simulink model "operationalSpaceInverseDynamicsControl"  (R2021a)
settings: Solver=VariableStepAuto  StartTime=0.0  StopTime=25  RelTol=1e-3
values from neighbouring files (symbols this model uses):
  Kd = diag([100, 100, 100, 50, 50, 50])    [assignment10_main.m]
  Kp = 5*diag([100, 100, 100,50,50,50])    [assignment10_main.m]
  x_d_const = [-0.139961 ... (first row only)    [assignment10_main.m]
libraries: vrlib x1, robotcorelib x1
settings Model: Creator=fabio  LastModifiedBy=fabio

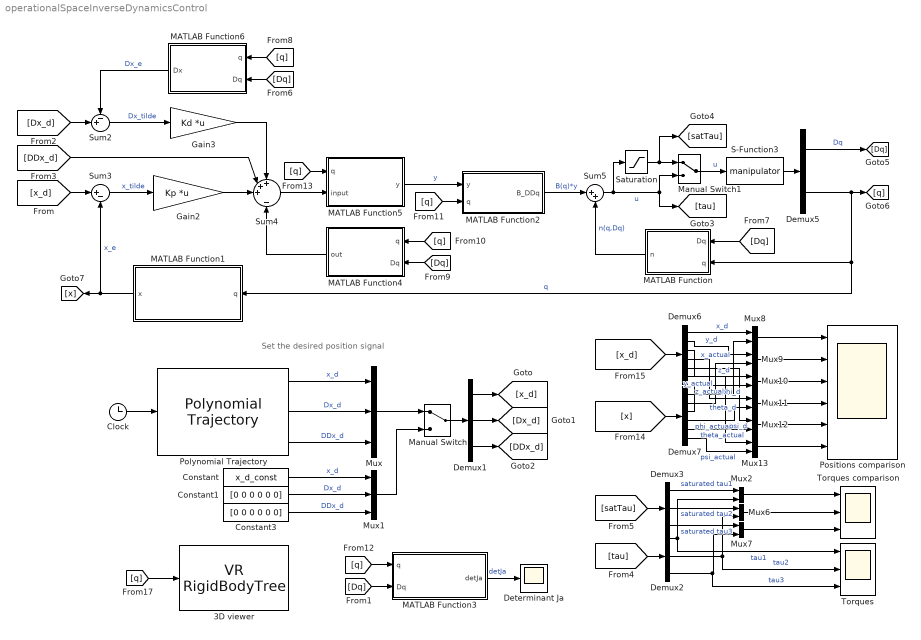
== system operationalSpaceInverseDynamicsControl ==
  note: Set the desired position signal
  3D viewer : vrlib/VR RigidBodyTree  RBT=robot  useRBT=off  Ts=0.5  ForceViewerOpen=on
      settings: SourceProductBaseCode=SL
  Clock : Clock
  Constant : Constant  Value=x_d_const
  Constant1 : Constant  Value=[0 0 0 0 0 0]
  Constant3 : Constant  Value=[0 0 0 0 0 0]
  Demux1 : Demux  Outputs=3
  Demux2 : Demux  Outputs=3
  Demux3 : Demux  Outputs=3
  Demux5 : Demux  Outputs=[3 3]
  Demux6 : Demux  Outputs=6
  Demux7 : Demux  Outputs=6
  Determinant Ja : Scope
  Gain2 : Gain  Gain=Kp  Multiplication=Matrix(K*u) (u vector)
  Gain3 : Gain  Gain=Kd  Multiplication=Matrix(K*u) (u vector)
  MATLAB Function : MATLAB Function  TreatAsAtomicUnit=on
  MATLAB Function1 : MATLAB Function  TreatAsAtomicUnit=on
  MATLAB Function2 : MATLAB Function  TreatAsAtomicUnit=on
  MATLAB Function3 : MATLAB Function  TreatAsAtomicUnit=on
  MATLAB Function4 : MATLAB Function  TreatAsAtomicUnit=on
  MATLAB Function5 : MATLAB Function  TreatAsAtomicUnit=on
  MATLAB Function6 : MATLAB Function  TreatAsAtomicUnit=on
  Manual Switch : ManualSwitch
  Manual Switch1 : ManualSwitch
  Mux : Mux  Inputs=3
  Mux1 : Mux  Inputs=3
  Mux{2,6..13} (9 alike) : Mux  Inputs=2
  Polynomial Trajectory : robotcorelib/Polynomial Trajectory  WaypointSource=Internal  Waypoints=x_d  TimePoints=[ 0, 10, 20]  TimeInterval=[ 1, 4 ]  Method=Cubic Polynomial  ParameterSource=Internal  VelocityBoundaryCondition=zeros( 6, 3)  AccelerationBoundaryCondition=zeros( 6, 3)  SimulateUsing=Interpreted execution
  Positions comparison : Scope  NumInputPorts=6
  S-Function3 : S-Function  FunctionName=manipulator  Parameters=myRobot  SFunctionDeploymentMode=off  EnableBusSupport=off
  Saturation : Saturate  UpperLimit=20  LowerLimit=-20
  Sum2 : Sum  Inputs=-+|
  Sum3 : Sum  Inputs=|+-
  Sum4 : Sum  Inputs=+++|-
  Sum5 : Sum  Inputs=|++
  Torques : Scope  NumInputPorts=3
  Torques comparison : Scope  NumInputPorts=3
  wires:
  Manual Switch1/1 -> S-Function3/1  "u"
  Sum3/1 -> Gain2/1  "x_tilde"
  S-Function3/1 -> Demux5/1
  Demux5/1 -> [Dq]  "Dq"
  Demux5/2 -> MATLAB Function1/1(q), MATLAB Function/2(q), [q]  "q"
  Gain2/1 -> Sum4/3
  Sum2/1 -> Gain3/1  "Dx_tilde"
  Gain3/1 -> Sum4/1
  Sum4/1 -> MATLAB Function5/2(input)
  MATLAB Function2/1(B_DDq) -> Sum5/1  "B(q)*y"
  MATLAB Function/1(n) -> Sum5/2  "n(q,Dq)"
  Clock/1 -> Polynomial Trajectory/1
  Polynomial Trajectory/2 -> Mux/2  "Dx_d"
  [DDx_d] -> Sum4/2
  [x_d] -> Sum3/1
  [Dx_d] -> Sum2/2
  Polynomial Trajectory/1 -> Mux/1  "x_d"
  Polynomial Trajectory/3 -> Mux/3  "DDx_d"
  Mux/1 -> Manual Switch/1
  Manual Switch/1 -> Demux1/1
  Demux1/1 -> [x_d]
  Demux1/2 -> [Dx_d]
  Demux1/3 -> [DDx_d]
  Constant/1 -> Mux1/1  "x_d"
  Constant1/1 -> Mux1/2  "Dx_d"
  Mux1/1 -> Manual Switch/2
  Constant3/1 -> Mux1/3  "DDx_d"
  Demux2/1 -> Torques/1, Mux2/2  "tau1"
  [tau] -> Demux2/1
  Saturation/1 -> [satTau], Manual Switch1/1
  [satTau] -> Demux3/1
  Demux3/1 -> Mux2/1  "saturated tau1"
  Mux2/1 -> Torques comparison/1
  Mux6/1 -> Torques comparison/2
  Mux7/1 -> Torques comparison/3
  Demux2/2 -> Torques/2, Mux6/2  "tau2"
  Demux3/2 -> Mux6/1  "saturated tau2"
  Demux3/3 -> Mux7/1  "saturated tau3"
  Demux2/3 -> Torques/3, Mux7/2  "tau3"
  Sum5/1 -> Manual Switch1/2, [tau], Saturation/1  "u"
  MATLAB Function1/1(x) -> Sum3/2, [x]  "x_e"
  [Dq] -> MATLAB Function/1(Dq)
  [Dq] -> MATLAB Function6/2(Dq)
  [q] -> MATLAB Function6/1(q)
  MATLAB Function6/1(Dx) -> Sum2/1  "Dx_e"
  [Dq] -> MATLAB Function4/2(Dq)
  [q] -> MATLAB Function4/1(q)
  MATLAB Function4/1(out) -> Sum4/4
  [q] -> MATLAB Function2/2(q)
  [q] -> MATLAB Function5/1(q)
  MATLAB Function5/1(y) -> MATLAB Function2/1(y)  "y"
  Demux6/2 -> Mux9/1  "y_d"
  Demux7/2 -> Mux9/2  "y_actual"
  [x_d] -> Demux6/1
  Demux6/5 -> Mux12/1  "theta_d"
  Demux7/1 -> Mux8/2  "x_actual"
  Demux6/4 -> Mux11/1  "phi_d"
  Demux7/4 -> Mux11/2  "phi_actual"
  Demux7/5 -> Mux12/2  "theta_actual"
  Demux7/6 -> Mux13/2  "psi_actual"
  Mux13/1 -> Positions comparison/6
  Mux9/1 -> Positions comparison/2
  Mux8/1 -> Positions comparison/1
  Mux10/1 -> Positions comparison/3
  [x] -> Demux7/1
  Demux6/1 -> Mux8/1  "x_d"
  Mux11/1 -> Positions comparison/4
  Demux7/3 -> Mux10/2  "z_actual"
  Demux6/6 -> Mux13/1  "psi_d"
  Mux12/1 -> Positions comparison/5
  Demux6/3 -> Mux10/1  "z_d"
  [q] -> 3D viewer/1
  [q] -> MATLAB Function3/1(q)
  [Dq] -> MATLAB Function3/2(Dq)
  MATLAB Function3/1(detJa) -> Determinant Ja/1  "detJa"

== matlab function operationalSpaceInverseDynamicsControl/MATLAB Function1 ==
  data: q input; x output
function x = k(q) 
    %Compute the direct kinematics from last transformation matrix
    if size(q,1) < 3
        q = [0 0 0];   
    end
    
    %get rotation matrix and translation vector from ∑0 to ∑ee   
    T0_to_ee = get_T0_ee_matrix(q);
    R0_to_ee = T0_to_ee(1:3,1:3);
    p0_to_ee = T0_to_ee(1:3,4);    
                 
    eulerAngles = rotm2eul(R0_to_ee, 'ZYZ');
  
    x = [ p0_to_ee;
          eulerAngles.' ]; %return complete direct kinematics
    
end

== matlab function operationalSpaceInverseDynamicsControl/MATLAB Function ==
  data: Dq input; n output; q input
function n = n_q_Dq(Dq, q)
    
    %To get the "perfect" matrices use the following code
    C = get_C_matrix(q,Dq);
    G = get_G_matrix(q);
    
    
    %To get the "wrongly estimated" matrices use the following code   
%     theta2 = q(2);   d3 = q(3); 
%     Dtheta2 = Dq(2); Dd3 = Dq(3); 
%     
%     m_Link4 = 0.16;  %0.2kg is the correct value
% 
%     C = [0,                         0,                        0;
%          0,            m_Link4*Dd3*d3,       m_Link4*Dtheta2*d3;
%          0,       -m_Link4*Dtheta2*d3,                        0];
%    
%     G = [           0                           ;
%          (981*m_Link4*sin(theta2)*d3)/100 ;
%           -(981*m_Link4*cos(theta2))/100    ];


    
    n = C*Dq + G; %F = friction is neglected

end

== matlab function operationalSpaceInverseDynamicsControl/MATLAB Function2 ==
  data: y input; B_DDq output; q input
function B_DDq = B_q(y,q)
    B_DDq = get_B_matrix(q)*y;
end

== matlab function operationalSpaceInverseDynamicsControl/MATLAB Function3 ==
  data: q input; detJa output; Dq input
function detJa = determinant_Ja(q, Dq)
    if size(q,1) < 3
        q = [0 0 0];   
    end  
    Ja = get_Ja_matrix(q);      
    detJa = det(Ja(1:3,1:3));
end

== matlab function operationalSpaceInverseDynamicsControl/MATLAB Function4 ==
  data: q input; out output; Dq input
function out = DJa_x_Dq(q, Dq)
    if size(q,1) < 3
        q = [0 0 0];   
    end  
    DJa = get_DJa_matrix(q, Dq);      
    out = DJa * Dq;
end

== matlab function operationalSpaceInverseDynamicsControl/MATLAB Function5 ==
  data: q input; y output; input input
function y = invJa(q, input)
    %Compute the numerical inverse analytical jacobian
    if size(q,1) < 3
        q = [0 0 0];   
    end  
    Ja = get_Ja_matrix(q);      
    
    y = pinv(Ja) * input;
 
end

== matlab function operationalSpaceInverseDynamicsControl/MATLAB Function6 ==
  data: q input; Dx output; Dq input
function Dx = Ja_x_Dq(q, Dq)
    if size(q,1) < 3
        q = [0 0 0];   
    end  
    Ja = get_Ja_matrix(q);      
    Dx = Ja * Dq;
end
